simulink library "csc_kfl_kalman_filter_mtv_lib"  (R2014b)
settings: Solver=ode45  SolverMode=SingleTasking  StartTime=0.0  StopTime=10.0  RelTol=1e-3
libraries: util_info_lib x1, csc_ekf_nonlinear_filter_mtv_lib x1, csc_snp_sensor_prep_mtv_lib x1
settings Model: ExtModeAutoUpdateStatusClock=off  Creator=Administrator  LastModifiedBy=mstewart

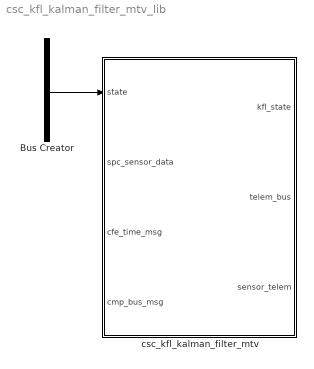
== system csc_kfl_kalman_filter_mtv_lib ==
  Bus Creator : BusCreator
  csc_kfl_kalman_filter_mtv : Subsystem
  wires:
  Bus Creator/1 -> csc_kfl_kalman_filter_mtv/1(state)
  ? -> Bus Creator/1  "x"
  ? -> Bus Creator/2  "accel"
  ? -> Bus Creator/3  "rate"
  ? -> Bus Creator/4  "q"

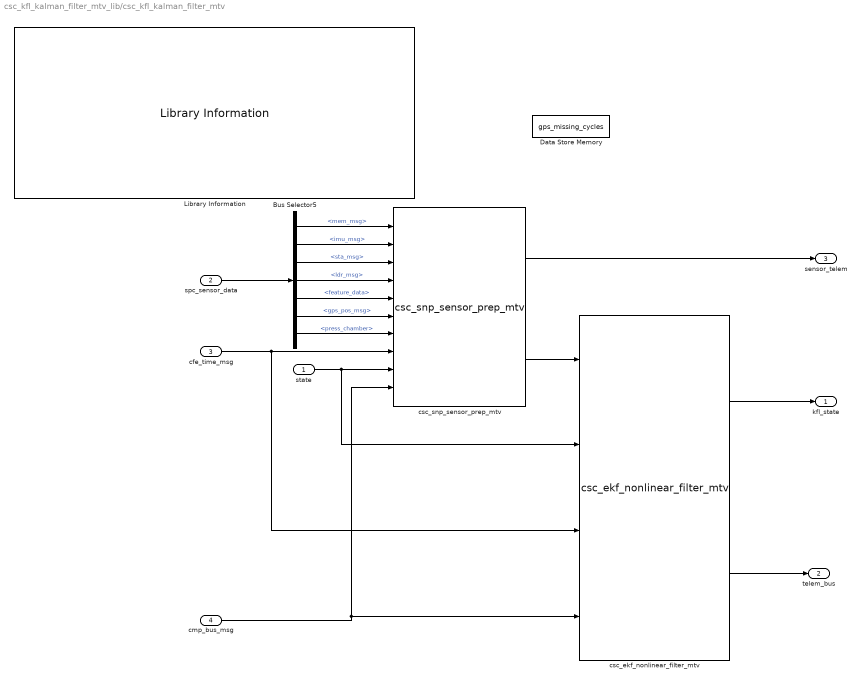
== system csc_kfl_kalman_filter_mtv_lib/csc_kfl_kalman_filter_mtv ==
  state : Inport
  spc_sensor_data : Inport  Port=2
  cfe_time_msg : Inport  Port=3
  cmp_bus_msg : Inport  Port=4
  Bus Selector5 : BusSelector  OutputSignals=mem_msg,imu_msg,sta_msg,ldr_msg,feature_data,gps_pos_msg,press_chamber
  Data Store Memory : DataStoreMemory  DataStoreName=gps_missing_cycles  ReadBeforeWriteMsg=warning  WriteAfterWriteMsg=warning  WriteAfterReadMsg=warning
  Library Information : util_info_lib/Library Information  owner='NONE'
  csc_ekf_nonlinear_filter_mtv : csc_ekf_nonlinear_filter_mtv_lib/csc_ekf_nonlinear_filter_mtv
  csc_snp_sensor_prep_mtv : csc_snp_sensor_prep_mtv_lib/csc_snp_sensor_prep_mtv
  kfl_state : Outport
  telem_bus : Outport  Port=2
  sensor_telem : Outport  Port=3
  wires:
  Bus Selector5/2 -> csc_snp_sensor_prep_mtv/2  "<imu_msg>"
  Bus Selector5/7 -> csc_snp_sensor_prep_mtv/7  "<press_chamber>"
  csc_snp_sensor_prep_mtv/1 -> sensor_telem/1
  Bus Selector5/6 -> csc_snp_sensor_prep_mtv/6  "<gps_pos_msg>"
  Bus Selector5/3 -> csc_snp_sensor_prep_mtv/3  "<sta_msg>"
  csc_ekf_nonlinear_filter_mtv/2 -> telem_bus/1
  Bus Selector5/1 -> csc_snp_sensor_prep_mtv/1  "<mem_msg>"
  Bus Selector5/5 -> csc_snp_sensor_prep_mtv/5  "<feature_data>"
  Bus Selector5/4 -> csc_snp_sensor_prep_mtv/4  "<ldr_msg>"
  spc_sensor_data/1 -> Bus Selector5/1
  csc_snp_sensor_prep_mtv/2 -> csc_ekf_nonlinear_filter_mtv/1
  cfe_time_msg/1 -> csc_snp_sensor_prep_mtv/8, csc_ekf_nonlinear_filter_mtv/3
  state/1 -> csc_snp_sensor_prep_mtv/9, csc_ekf_nonlinear_filter_mtv/2
  csc_ekf_nonlinear_filter_mtv/1 -> kfl_state/1
  cmp_bus_msg/1 -> csc_ekf_nonlinear_filter_mtv/4, csc_snp_sensor_prep_mtv/10
